simulink model "gamma_correction"  (R2016a)
settings: Solver=VariableStepAuto  StartTime=0.0  StopTime=Inf  RelTol=1e-3
PreLoadFcn:
  | gamma = 0.45
libraries: visionsinks x3, dspvision x1, ModelComposer x1
settings Model: Creator=ukumar  LastModifiedBy=wesleyl

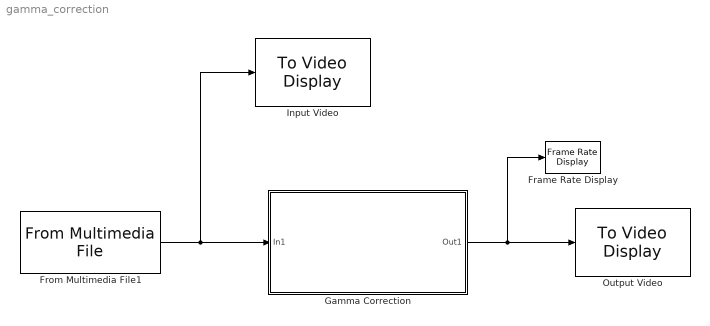
== system gamma_correction ==
  Frame Rate Display : visionsinks/Frame Rate Display  UpdateRate=10
  From Multimedia File1 : dspvision/From Multimedia File  inputFilename=handshake_left.avi  loop=on  numPlays=inf  outputStreams=Video only  videoDataType=uint8  audioDataType=int16  inheritSampleTime=off  userDefinedSampleTime=1/30  noAudioOutput=off  isIntensityVideo=off  fourcc=Intensity  colorVideoFormat=One multidimensional signal  outputEOF=off  dataOrg=Column-major  audioFrameSize=1024  computeAudioFrameSize=off  outSamplingMode=Sample based
  Gamma Correction : Subsystem
  Input Video : visionsinks/To Video Display  windowSizeMode=True size (1:1)  openAtMdlStart=on  fullScreen=off  videoWindowX=34  videoWindowY=182  saveWindowSize=off  videoWindowWidth=640  videoWindowHeight=480  inputColorFormat=RGB  inputType=Obsolete  imagePorts=One multidimensional signal  OutputDevice=On-screen video monitor  dataOrg=Column-major  isWindowOpen=off
  Output Video : visionsinks/To Video Display  windowSizeMode=True size (1:1)  openAtMdlStart=on  fullScreen=off  videoWindowX=566  videoWindowY=180  saveWindowSize=off  videoWindowWidth=640  videoWindowHeight=480  inputColorFormat=RGB  inputType=Obsolete  imagePorts=One multidimensional signal  OutputDevice=On-screen video monitor  dataOrg=Column-major  isWindowOpen=off
  wires:
  From Multimedia File1/1 -> Gamma Correction/1(In1), Input Video/1
  Gamma Correction/1(Out1) -> Frame Rate Display/1, Output Video/1

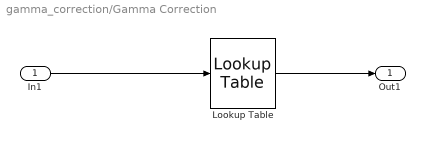
== system gamma_correction/Gamma Correction ==
  In1 : Inport
  Lookup Table : ModelComposer/Lookup Table  Description=Performs table look-up  TableData=(([0:255]/255).^gamma)*255  TableBias=0  WrapAround=Saturate at table ends  OutDataType=uint8  TypeExp=''  Signedness=Signed  WordLength=16  FractionalLength=10  RoundingMode=Truncation to minus infinity  OverflowMode=Wrap around
  Out1 : Outport
  wires:
  Lookup Table/1 -> Out1/1
  In1/1 -> Lookup Table/1
